simulink model "gmp_pmsm_sil"  (R2022b)
settings: Solver=VariableStepAuto  StartTime=0.0  StopTime=2.5  RelTol=1e-3
libraries: peripheral_utilities x2, spsControlledVoltageSourceLib x1, gmp_sil_core_pack x1, spsPermanentMagnetSynchronousMachineLib x1, spspowerguiLib x1
settings Model: SimulationMode=accelerator  Creator=javnson  LastModifiedBy=javnson

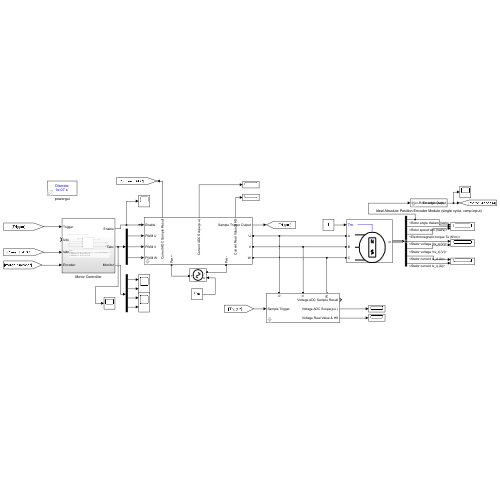
[thumbnail: Simulink's stored preview of the top-level diagram]
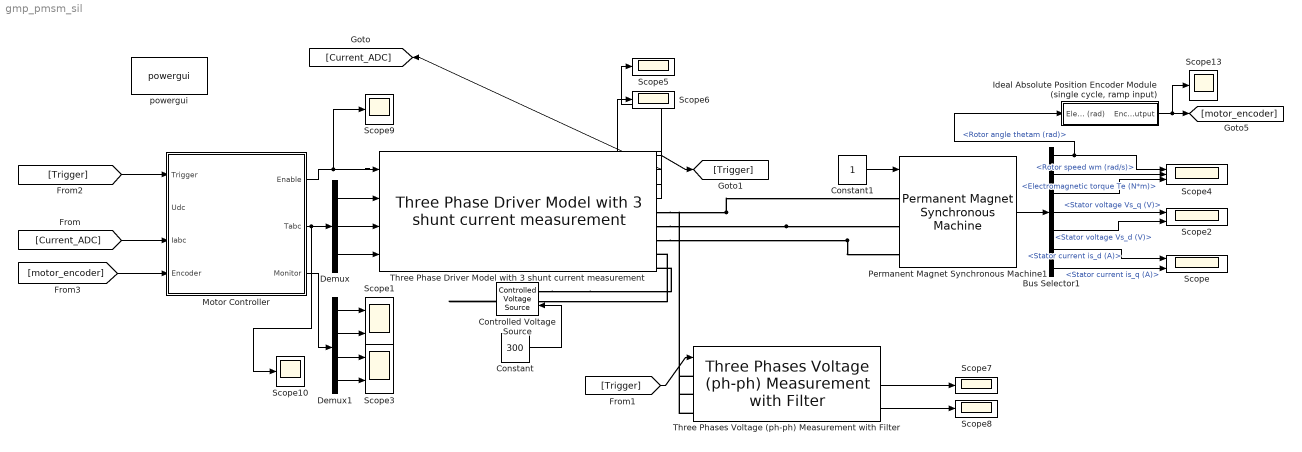
== system gmp_pmsm_sil ==
  Bus Selector1 : BusSelector  OutputSignals=Rotor angle thetam (rad),Rotor speed wm (rad/s),Electromagnetic torque Te (N*m),Stator voltage Vs_q (V),Stator voltage Vs_d (V),Stator current is_d (A),Stator current is_q (A)
  Constant : Constant  Value=300
  Constant1 : Constant
  Controlled Voltage Source : spsControlledVoltageSourceLib/Controlled Voltage Source  Initialize=on  Source_Type=AC  Amplitude=0  Phase=0  Frequency=0  Measurements=None
  Demux : Demux  Outputs=3
  Demux1 : Demux
  "Ideal Absolute Position Encoder Module (single cycle, ramp input)" : Subsystem  mask{ENCODER_BIT=17}
      mask DialogControl DescGroupVar Prompt: Ideal Absolute Position Encoder Module (single cycle)
      mask DialogControl DescTextVar Prompt: Avsolute Encoder transfer a motor mechanical angle (thetam, rad) to Absolute Encoder result. Generally, an absolute encoder has 17-bits or 23-bits resolution results.
      mask DialogControl ParameterGroupVar Prompt: 参数
      mask DialogControl Control2 Prompt: Absolute Encoder Resolution (bits):
  Motor Controller : Subsystem
  Permanent Magnet Synchronous Machine1 : spsPermanentMagnetSynchronousMachineLib/Permanent Magnet Synchronous Machine  NbPhases=3  FluxDistribution=Sinusoidal  RotorType=Round  MechanicalLoad=Torque Tm  PresetModel=No  ShowDetailedParameters=on  MeasurementBus=off  Resistance=2.875  Inductance=8.5e-3  dqInductances=[8.5e-3,8.5e-3]  La=0.00835  MachineConstant=Flux linkage established by magnets (V.s)  Flux=0.22  VoltageCst=39.9036  TorqueCst=0.33  Flat=120  Mechanical=[0.005 0.003 1 0]  PolePairs=4  InitialConditions=[0, 0, 0, 0]  InitialConditions5ph=[0 0 0 0 0 0]  RefAngle=Aligned with phase A axis (original Park)  IterativeDiscreteModel=Trapezoidal non iterative  TsBlock=-1  TsPowergui=0
  Scope{,1..3} (4 alike) : Scope  NumInputPorts=2
  Scope{5..10,13} (7 alike) : Scope
  Scope4 : Scope  NumInputPorts=3
  Three Phase Driver Model with 3 shunt current measurement : peripheral_utilities/Three Phase Driver Model with 3 shunt current measurement  fswitch=10e3  CMP_MAX=10000  Deadband_Upper=200  Deadband_Lower=200  Deadband_us=2  phase_shift=0  R_mosfet_on=0.1  Lon=0  Rd=0.01  Vf=0.3  Rs=1e5  Cs=inf  Rsap=0.02  ADC_GAIN=1  ADC_BIT=16  ADC_REFERENCE=3.3  ADC_BIAS=1.5  ADC_INIT=0
      settings: SourceProductName=GMP Utilities Library
  Three Phases Voltage (ph-ph) Measurement with Filter : peripheral_utilities/Three Phases Voltage (ph-ph) Measurement with Filter  ADC_GAIN=1  ADC_BIT=16  ADC_REFERENCE=600  ADC_BIAS=300  ADC_INIT=0  cut_frequency=500
      settings: SourceProductName=GMP Utilities Library
  powergui : spspowerguiLib/powergui  Priority=1  SimulationMode=Discrete  SampleTime=1e-7  frequency=60  Iterations=50  frequencyindice=0  Pbase=100e6  ErrMax=1e-4  UnitsV=kV  UnitsW=MW  buscounter=0  FunctionMessages=off  echomessages=off  EnableUseOfTLC=off  CurrentSourceSwitches=off  DisableSnubberDevices=off  DisableRonSwitches=off  DisableVfSwitches=off  DisplayEquations=off  AutomaticDiscreteSolvers=off  SolverType=Tustin/Backward Euler (TBE)  Interpol=off  ExternalGateDelay=off  methode=off  Ts=100  x0status=blocks  SPID=on  SwTol=0  HookPort=off  NonlinearTolerance=1e-4  nMaxIteration=100  ContinueOnMaxIteration=off  RestoreLinks=warning  ResistiveCurrentMeasurement=off  Frange=[0:2:500]  Ylog=off  Xlog=on  ShowGrid=off  save=off  variable=ZData  structure=0  ZoomFFT=off  StartTime=0.0  cycles=1  DisplayStyle=1  fundamental=60  FreqAxis=off  MaxFrequency=1000  frequencyindicesteady=1  RmsSteady=1  display=off
  wires:
  Motor Controller/1(Enable) -> Scope9/1, Three Phase Driver Model with 3 shunt current measurement/1
  Demux/1 -> Three Phase Driver Model with 3 shunt current measurement/2
  Demux/2 -> Three Phase Driver Model with 3 shunt current measurement/3
  Demux/3 -> Three Phase Driver Model with 3 shunt current measurement/4
  Motor Controller/2(Tabc) -> Demux/1, Scope10/1
  Constant/1 -> Controlled Voltage Source/1
  Bus Selector1/4 -> Scope2/1  "<Stator voltage Vs_q (V)>"
  Bus Selector1/5 -> Scope2/2  "<Stator voltage Vs_d (V)>"
  Bus Selector1/2 -> Scope4/2  "<Rotor speed wm (rad/s)>"
  "Ideal Absolute Position Encoder Module (single cycle, ramp input)"/1(Encoder Output) -> Scope13/1, [motor_encoder]
  Bus Selector1/1 -> Scope4/1, "Ideal Absolute Position Encoder Module (single cycle, ramp input)"/1(Elec-Rotor angle (rad))  "<Rotor angle thetam (rad)>"
  Bus Selector1/3 -> Scope4/3  "<Electromagnetic torque Te (N*m)>"
  Permanent Magnet Synchronous Machine1/1 -> Bus Selector1/1
  Bus Selector1/6 -> Scope/1  "<Stator current is_d (A)>"
  Bus Selector1/7 -> Scope/2  "<Stator current is_q (A)>"
  Three Phase Driver Model with 3 shunt current measurement/2 -> [Current_ADC]
  [Current_ADC] -> Motor Controller/3(Iabc)
  Three Phase Driver Model with 3 shunt current measurement/1 -> [Trigger]
  [Trigger] -> Three Phases Voltage (ph-ph) Measurement with Filter/1
  [Trigger] -> Motor Controller/1(Trigger)
  [motor_encoder] -> Motor Controller/4(Encoder)
  Motor Controller/3(Monitor) -> Demux1/1
  Demux1/1 -> Scope1/1
  Demux1/2 -> Scope1/2
  Demux1/3 -> Scope3/1
  Demux1/4 -> Scope3/2
  Constant1/1 -> Permanent Magnet Synchronous Machine1/1
  Three Phase Driver Model with 3 shunt current measurement/3 -> Scope5/1
  Three Phase Driver Model with 3 shunt current measurement/4 -> Scope6/1
  Three Phases Voltage (ph-ph) Measurement with Filter/2 -> Scope7/1
  Three Phases Voltage (ph-ph) Measurement with Filter/3 -> Scope8/1
  connections:
  Controlled Voltage Source/RConn1 -- Three Phase Driver Model with 3 shunt current measurement/RConn4
  Controlled Voltage Source/LConn1 -- Three Phase Driver Model with 3 shunt current measurement/RConn5
  Three Phase Driver Model with 3 shunt current measurement/RConn1 -- Permanent Magnet Synchronous Machine1/LConn1 -- Three Phases Voltage (ph-ph) Measurement with Filter/LConn1
  Three Phase Driver Model with 3 shunt current measurement/RConn2 -- Three Phases Voltage (ph-ph) Measurement with Filter/LConn2 -- Permanent Magnet Synchronous Machine1/LConn2
  Three Phase Driver Model with 3 shunt current measurement/RConn3 -- Three Phases Voltage (ph-ph) Measurement with Filter/LConn3 -- Permanent Magnet Synchronous Machine1/LConn3

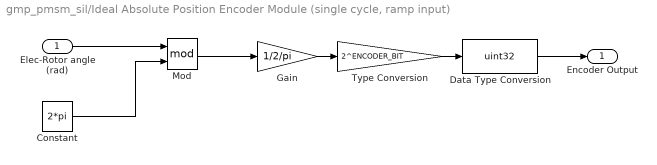
== system gmp_pmsm_sil/Ideal Absolute Position Encoder Module (single cycle, ramp input) ==
  Elec-Rotor angle (rad) : Inport
  Constant : Constant  Value=2*pi
  Data Type Conversion : DataTypeConversion  OutDataTypeStr=uint32  SaturateOnIntegerOverflow=off  RndMeth=Floor
  Gain : Gain  Gain=1/2/pi
  Mod : Math  Operator=mod
  Type Conversion : Gain  Gain=2^ENCODER_BIT
  Encoder Output : Outport
  wires:
  Gain/1 -> Type Conversion/1
  Type Conversion/1 -> Data Type Conversion/1
  Data Type Conversion/1 -> Encoder Output/1
  Elec-Rotor angle (rad)/1 -> Mod/1
  Mod/1 -> Gain/1
  Constant/1 -> Mod/2

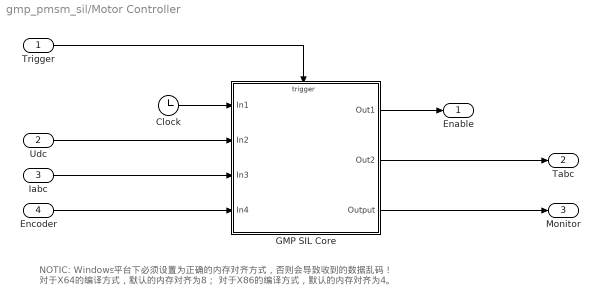
== system gmp_pmsm_sil/Motor Controller ==
  note: NOTIC:
      | Windows平台下必须设置为正确的内存对齐方式，否则会导致收到的数据乱码！
      | 对于X64的编译方式，默认的内存对齐为8；
      | 对于X86的编译方式，默认的内存对齐为4。
  Trigger : Inport
  Udc : Inport  Port=2
  Iabc : Inport  Port=3
  Encoder : Inport  Port=4
  Clock : Clock
  GMP SIL Core : Subsystem
  Enable : Outport
  Tabc : Outport  Port=2
  Monitor : Outport  Port=3
  wires:
  Clock/1 -> GMP SIL Core/1(In1)
  Udc/1 -> GMP SIL Core/2(In2)
  Iabc/1 -> GMP SIL Core/3(In3)
  GMP SIL Core/1(Out1) -> Enable/1
  GMP SIL Core/2(Out2) -> Tabc/1
  Trigger/1 -> GMP SIL Core/Trigger
  Encoder/1 -> GMP SIL Core/4(In4)
  GMP SIL Core/3(Output) -> Monitor/1

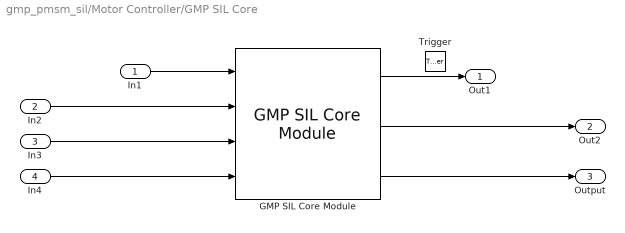
== system gmp_pmsm_sil/Motor Controller/GMP SIL Core ==
  In1 : Inport
  In2 : Inport  Port=2
  In3 : Inport  Port=3
  In4 : Inport  Port=4
  Trigger : TriggerPort  VariantControl=(inherit)  PortDimensions=1
  GMP SIL Core Module : gmp_sil_core_pack/GMP SIL Core Module  MaskPackedDataTypes={'double','uint32','uint32', 'uint32'}  MaskPackedDataSizes={[1],[1],[3],[1]}  MaskUnpackedDataTypes={'uint32','uint32','double'}  MaskUnpackedDataSizes={[1],[3],[4]}  MaskAlignment=1  MaskHostAddr='127.0.0.1'  MaskMsgTxPort=12300  MaskMsgRxPort=12301  MaskCmdTxPort=12302  MaskCmdRxPort=12303
      settings: SourceProductName=GMP Utilities Library
  Out1 : Outport
  Out2 : Outport  Port=2
  Output : Outport  Port=3
  wires:
  GMP SIL Core Module/1 -> Out1/1
  In1/1 -> GMP SIL Core Module/1
  In2/1 -> GMP SIL Core Module/2
  In3/1 -> GMP SIL Core Module/3
  GMP SIL Core Module/2 -> Out2/1
  In4/1 -> GMP SIL Core Module/4
  GMP SIL Core Module/3 -> Output/1
